simulink model "Long_Calibrate"  (R2020b)
settings: Solver=VariableStepAuto  StartTime=0.0  StopTime=60  RelTol=1e-3
values from neighbouring files (symbols this model uses):
  Accreq_valueY = [-6 -5.8 -5.6 -5.4 -5.2 -5 -4.8 -4.6 -4.4 -4.2 -4 -3.8 ... (53 elements, 1x53)]    [Accreq_valueY.mat]    (also in make_calibrate_table.m = [-6:0.2:-0.1,0.1:0.2:4.5])
  Openness_valueZ = [-100 -100 -100 -100 -96.0255330412 -92.5475086479 -89.5294536846 -86.0415379146 -82.7286102821 -79.845577645 -76.1908087806 -72.5393369095 ... (1643 elements, 53x31)]    [Openness_valueZ.mat]    (also in make_calibrate_table.m = zeros(length(Accreq_valueY), length(Vehspd_valueX)))
  Vehspd_valueX = [0 4 8 12 16 20 24 28 32 36 40 44 ... (31 elements, 1x31)]    [Vehspd_valueX.mat]    (also in make_calibrate_table.m = 0:4:120)
libraries: Solver_SF x1, simulink x1
settings Model: Creator=cv  LastModifiedBy=cv

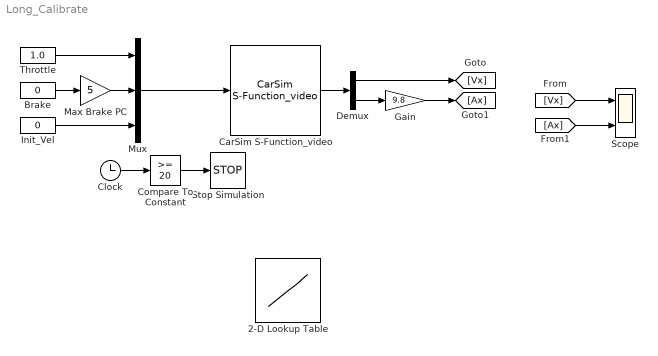
== system Long_Calibrate ==
  2-D Lookup Table : Lookup_n-D  BreakpointsForDimension1=Accreq_valueY  BreakpointsForDimension2=Vehspd_valueX  Table=Openness_valueZ  InternalRulePriority=Speed  RndMeth=Simplest  InputSameDT=on
      settings: InputPortMap=u0,u1
  Brake : Constant  Value=0
  CarSim S-Function_video : Solver_SF/CarSim S-Function_video  Priority=1  SIMFILE=calibrated.sim
      settings: SourceProductName=CarSim S-Function
  Clock : Clock
  Compare To Constant : simulink/Logic and Bit Operations/Compare To Constant  relop=>=  const=20  OutDataTypeStr=boolean
  Demux : Demux  Outputs=2
  Gain : Gain  Gain=9.8
  Init_Vel : Constant  Value=0
  Max Brake PC : Gain  Gain=5
  Mux : Mux  Inputs=3
  Scope : Scope  NumInputPorts=2
  Stop Simulation : Stop
  Throttle : Constant  Value=1.0
  wires:
  Mux/1 -> CarSim S-Function_video/1
  CarSim S-Function_video/1 -> Demux/1
  Demux/1 -> [Vx]
  Demux/2 -> Gain/1
  Gain/1 -> [Ax]
  Throttle/1 -> Mux/1
  Brake/1 -> Max Brake PC/1
  [Vx] -> Scope/1
  [Ax] -> Scope/2
  Max Brake PC/1 -> Mux/2
  Init_Vel/1 -> Mux/3
  Clock/1 -> Compare To Constant/1
  Compare To Constant/1 -> Stop Simulation/1
